simulink library "lib_energy_storage"  (Simulink 7.9)
settings: Solver=ode45  SolverMode=SingleTasking  StartTime=0.0  StopTime=10.0  RelTol=1e-3
undefined symbols (not defined in the file or in its folder): air_cp, amb_tmp, cyc_mph, enable_stop, ess_cap, ess_cap_scale, ess_cb, ess_cc, ess_coulombic_eff, ess_init_soc, ess_max_ah_cap, ess_max_p, ess_max_p_soc, ess_max_soc, ess_max_volts, ess_min_soc, ess_min_volts, ess_MMi, ess_MMo, ess_mod_airflow, ess_mod_cp, ess_mod_cpm, ess_mod_init_tmp, ess_module_mass, ess_module_num, ess_on, ess_parallel_mod_num, ess_r, ess_r_chg, ess_r_dis, ess_rc, ess_re, ess_res_scale_coef, ess_res_scale_fun, ess_rt, ess_set_tmp, ess_soc, ess_th_calc, ess_th_res, ess_th_res_off, ess_th_res_on, ess_tmp, ess_voc, fund_byu, fund_byuop, mc_min_volts, saber_air_temp, Saber_Battery_IO_File, saber_init_soc, saber_init_temp, saber_init_voc, saber_k_cb, saber_k_cc, saber_k_rc, saber_k_re, saber_k_rt, saber_k_soc, t_soc, time_step
libraries: lib_energy_storage x3
(part 1 of 3)
Description:
  | energy storage
settings Model: Creator=NREL  LastModifiedBy=mokeefe  ModifiedComment=mzolot -- Mon Apr 29 15:28:23 2002 -- Version 3.0107
settings Model: ModifiedHistory=|
  | mzolot -- Mon Apr 29 15:28:23 2002 -- Version 3.0107
  | 
  | 
  | mzolot -- Mon Apr 29 15:28:23 2002 -- Version 3.0107
  | 
  | 
  | mzolot -- Mon Apr 29 15:09:57 2002 -- Version 3.0106
  | 
  | 
  | mzolot -- Mon Apr 29 14:58:03 2002 -- Version 3.0105
  | 
  | 
  | mzolot -- Mon Apr 29 14:03:19 2002 -- Version 3.0104
  | 
  | 
  | mzolot -- Mon Apr 29 14:02:44 2002 -- Version 3.0103
  | 
  | 
  | mzolot -- Mon Apr 29 14:02:36 2002 -- Version 3.0102
  | 
  | 
  | mzolot -- Mon Apr 29 14:01:30 2002 -- Version 3.0101
  | 
  | 
  | mzolot -- Tue Apr 23 09:34:07 2002 -- Version 3.0100
  | 
  | 
  | mzolot -- Tue Apr 23 09:26:47 2002 -- Version 3.099
  | 
  | 
  | mzolot -- Tue Apr 23 09:26:41 2002 -- Version 3.098
  | 
  | 
  | mzolot -- Fri Apr 19 16:37:41 2002 -- Version 3.097
  | 
  | 
  | mzolot -- Fri Apr 19 11:13:38 2002 -- Version 3.096
  | 
  | 
  | mzolot -- Thu Apr 18 17:16:22 2002 -- Version 3.095
  | 
  | 
  | mokeefe -- Thu Apr 18 08:28:08 2002 -- Version 3.094
  | saving the model:
  | o "without the model browser open"
  | o with only top-level screen visible
  | o with "fit to view" enabled
  | o with "status bar" off and "toolbar" off
  | o with "prompt to update model history with each save" on
  | 
  | vjohnson -- Thu Jan 25 10:35:56 2001 -- Version 3.02
  | 
  | 
  | ssprik -- Wed Nov 01 15:28:33 2000 -- Version 3.01
  | enabled comment dialogue to prompt the person saving the model to add comments.

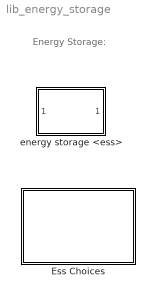
== system lib_energy_storage ==
  note: Energy Storage:
  Ess Choices : Subsystem
  energy storage <ess> : Subsystem  AncestorBlock=lib_energy_storage/Subsystem/energy storage <ess>
      mask Display: image(imread('bdi_ess.jpg'))

== system lib_energy_storage/Ess Choices ==
  note: Nnet
  note: Fundamental
  note: Saber Cosim
  Ultracapacitor  System : Subsystem
      mask Display: image(imread('bdi_ess.jpg'))
  energy storage <ess> : Subsystem
      mask Display: image(imread('bdi_ess.jpg'))
  energy storage <ess> RC : Subsystem
      mask Display: image(imread('bdi_ess.jpg'))
  energy storage <ess> nnet : Subsystem
      mask Display: image(imread('bdi_ess.jpg'))
  energy storage <ess> Saber : Subsystem
      mask Display: image(imread('bdi_ess.jpg'))
  energy storage <ess> fundamental model : Subsystem
      mask Display: image(imread('bdi_ess.jpg'))
  energy storage <ess> optima fundamental model : Subsystem
      mask Display: image(imread('bdi_ess.jpg'))
  ess config : Subsystem  BlockChoice="Ultracapacitor  System"
      settings: TemplateBlock=self  MemberBlocks="Ultracapacitor  System,energy storage <ess>,energy storage <ess> RC,energy storage <ess> nnet,energy storage <ess> Saber,energy storage <ess> fundamental model,energy storage <ess> optima fundamental model"

== system lib_energy_storage/energy storage <ess> ==
  power req'd into bus (W) : Inport
  ess config : Subsystem  BlockChoice="Ultracapacitor  System"
      settings: AttributesFormatString=%<BlockChoice>  TemplateBlock=lib_energy_storage/Ess Choices/ess config  MemberBlocks="Ultracapacitor  System,energy storage <ess>,energy storage <ess> RC,energy storage <ess> nnet,energy storage <ess> Saber,energy storage <ess> fundamental model,energy storage <ess> optima fundamental model"
  power available to bus (W) : Outport  InitialOutput=0
  wires:
  ess config/1(power available to bus (W)) -> power available to bus (W)/1
  power req'd into bus (W)/1 -> ess config/1(power req'd into bus (W))

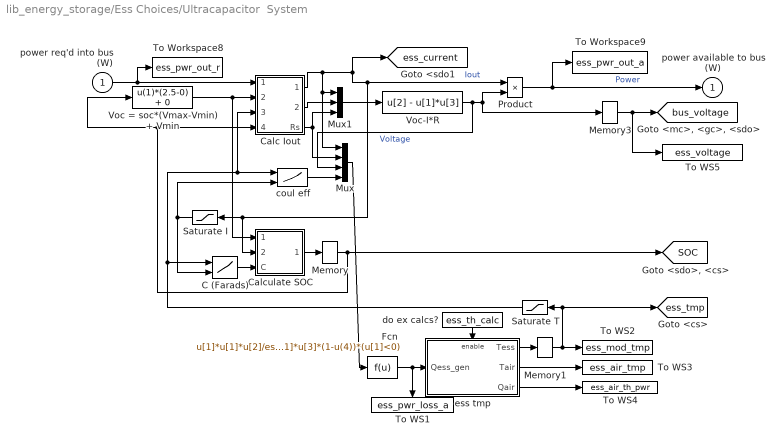
== system lib_energy_storage/Ess Choices/Ultracapacitor  System ==
  power req'd into bus (W) : Inport
  C (Farads) : Lookup2D  RowIndex=ess_tmp  ColumnIndex=ess_i  Table=ess_cap  SaturateOnIntegerOverflow=on  InputSameDT=on
  Calc Iout : Subsystem
  Calculate SOC : Subsystem
  Fcn : Fcn  Expr=u[1]*u[1]*u[2]/ess_parallel_mod_num*(u[1]>=0)+u[1]*u[1]*u(4)*u(4)*u[2]/ess_parallel_mod_num*(u[1]<0)-u[1]*u[3]*(1-u(4))*(u[1]<0)
  Memory : Memory  X0=ess_init_soc
  Memory1 : Memory  X0=ess_mod_init_tmp
  Memory3 : Memory  X0=(ess_init_soc*(2.5-0)+0)*ess_module_num
  Mux : Mux
  Mux1 : Mux  Inputs=3
  Product : Product  SaturateOnIntegerOverflow=on  RndMeth=Zero  InputSameDT=on  OutDataTypeStr=Inherit: Same as first input
  Saturate I : Saturate  UpperLimit=225  LowerLimit=-225
  Saturate T : Saturate  UpperLimit=40  LowerLimit=0
  To WS1 : ToWorkspace  VariableName=ess_pwr_loss_a
  To WS2 : ToWorkspace  VariableName=ess_mod_tmp
  To WS3 : ToWorkspace  VariableName=ess_air_tmp
  To WS4 : ToWorkspace  VariableName=ess_air_th_pwr
  To WS5 : ToWorkspace  VariableName=ess_voltage
  To Workspace8 : ToWorkspace  VariableName=ess_pwr_out_r  SampleTime=-1
  To Workspace9 : ToWorkspace  VariableName=ess_pwr_out_a  SampleTime=-1
  Voc = soc*(Vmax-Vmin) + Vmin : Fcn  Expr=u(1)*(2.5-0) + 0
  Voc-I*R : Fcn  Expr=u[2] - u[1]*u[3]
  coul eff : Lookup2D  RowIndex=ess_tmp  ColumnIndex=ess_i  Table=ess_coulombic_eff  SaturateOnIntegerOverflow=on  InputSameDT=on
  do ex calcs? : Constant  Value=ess_th_calc
  ess tmp : Subsystem  TreatAsAtomicUnit=on
  power available to bus (W) : Outport  InitialOutput=0
  tag scope: SOC=global, bus_voltage=global, ess_current=global, ess_tmp=global
  wires:
  power req'd into bus (W)/1 -> Calc Iout/1(Preq), To Workspace8/1
  Memory/1 -> [SOC], Voc = soc*(Vmax-Vmin) + Vmin/1, Calc Iout/4(SOC)
  Product/1 -> power available to bus (W)/1, To Workspace9/1  "Power"
  Calc Iout/1(Iout) -> Mux/1, Mux1/1, Product/1, Calculate SOC/2(Iout), Saturate I/1, [ess_current]  "Iout"
  coul eff/1 -> Mux/4
  Mux/1 -> Fcn/1
  Mux1/1 -> Voc-I*R/1
  Calc Iout/3(Rs) -> Mux/2, Mux1/3
  Fcn/1 -> ess tmp/1(Qess_gen), To WS1/1
  do ex calcs?/1 -> ess tmp/Enable
  ess tmp/1(Tess) -> Memory1/1
  ess tmp/2(Tair) -> To WS3/1
  Memory1/1 -> [ess_tmp], To WS2/1, Saturate T/1
  ess tmp/3(Qair) -> To WS4/1
  Voc-I*R/1 -> Product/2, Memory3/1, Mux/3  "Voltage"
  Memory3/1 -> [bus_voltage], To WS5/1
  Calculate SOC/1(SOC) -> Memory/1
  C (Farads)/1 -> Calculate SOC/3(C)
  Voc = soc*(Vmax-Vmin) + Vmin/1 -> Calc Iout/2(Voc), Calculate SOC/1(Voc)
  Saturate I/1 -> C (Farads)/2, coul eff/2
  Calc Iout/2(Voc*k) -> Mux1/2
  Saturate T/1 -> C (Farads)/1, coul eff/1, Calc Iout/3(tmp)

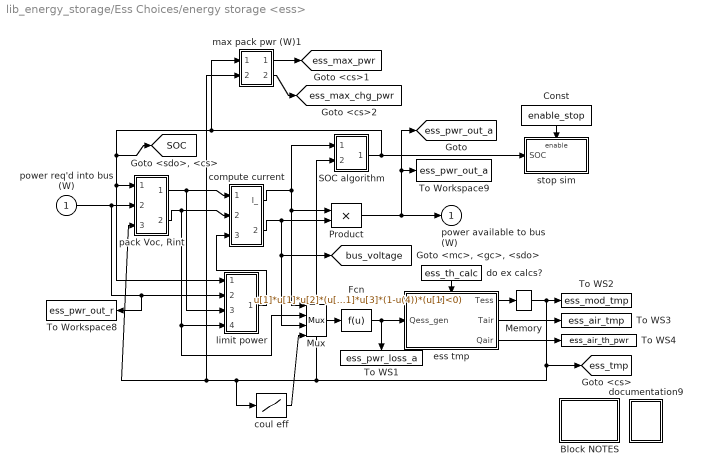
== system lib_energy_storage/Ess Choices/energy storage <ess> ==
  power req'd into bus (W) : Inport
  Block NOTES : Subsystem
      mask Display: disp('Block\nNOTES')
  Const : Constant  Value=enable_stop
  Fcn : Fcn  Expr=u[1]*u[1]*u[2]*(u[1]>=0)+u[1]*u[1]*u[2]*u(4)*u(4)*(u[1]<0)-u[1]*u[3]*(1-u(4))*(u[1]<0)
  Memory : Memory  X0=ess_mod_init_tmp
  Mux : Mux
  Product : Product  SaturateOnIntegerOverflow=on  RndMeth=Zero  InputSameDT=on  OutDataTypeStr=Inherit: Same as first input
  SOC algorithm : Subsystem
  To WS1 : ToWorkspace  VariableName=ess_pwr_loss_a
  To WS2 : ToWorkspace  VariableName=ess_mod_tmp
  To WS3 : ToWorkspace  VariableName=ess_air_tmp
  To WS4 : ToWorkspace  VariableName=ess_air_th_pwr
  To Workspace8 : ToWorkspace  VariableName=ess_pwr_out_r  SampleTime=-1
  To Workspace9 : ToWorkspace  VariableName=ess_pwr_out_a  SampleTime=-1
  compute current : Subsystem
  coul eff : Lookup  InputValues=ess_tmp  Table=ess_coulombic_eff  SaturateOnIntegerOverflow=on
  do ex calcs? : Constant  Value=ess_th_calc
  documentation9 : Subsystem
      settings: OpenFcn=web(['file:\\\' which('energy_storage.htm')]);
      mask Display: image(imread('doc_man.jpg'))
  ess tmp : Subsystem  TreatAsAtomicUnit=on
  limit power : Subsystem
  max pack pwr (W)1 : Subsystem
  "pack Voc, Rint" : Subsystem
  stop sim : Subsystem  TreatAsAtomicUnit=on
  power available to bus (W) : Outport  InitialOutput=0
  tag scope: SOC=global, bus_voltage=global, ess_max_chg_pwr=global, ess_max_pwr=global, ess_pwr_out_a=global, ess_tmp=global
  wires:
  compute current/2(V_) -> Product/2, Mux/3, [bus_voltage]
  Mux/1 -> Fcn/1
  power req'd into bus (W)/1 -> To Workspace8/1, limit power/2(Pbty), "pack Voc, Rint"/2(req'd battery power (W))
  compute current/1(I_) -> SOC algorithm/1((A)), Product/1, Mux/1
  Product/1 -> power available to bus (W)/1, To Workspace9/1, [ess_pwr_out_a]
  Fcn/1 -> To WS1/1, ess tmp/1(Qess_gen)
  do ex calcs?/1 -> ess tmp/Enable
  SOC algorithm/1(SOC1) -> stop sim/1(SOC), [SOC], "pack Voc, Rint"/1(SOC (prev)), limit power/1(SOC), max pack pwr (W)1/1(SOC)
  Const/1 -> stop sim/Enable
  "pack Voc, Rint"/2(pack resistance) -> compute current/2(Rint), limit power/4(Rint), Mux/2
  "pack Voc, Rint"/1(pack open- circuit voltage) -> compute current/1(Voc), limit power/3(Voc)
  limit power/1("Pbty, limited") -> compute current/3(limited output power (W))
  ess tmp/2(Tair) -> To WS3/1
  ess tmp/3(Qair) -> To WS4/1
  ess tmp/1(Tess) -> Memory/1
  coul eff/1 -> Mux/4
  max pack pwr (W)1/1(max ess discharge pwr) -> [ess_max_pwr]
  Memory/1 -> To WS2/1, SOC algorithm/2(tmp (C)), coul eff/1, "pack Voc, Rint"/3(mod tmp   (C)), max pack pwr (W)1/2(ess_mod_tmp), [ess_tmp]
  max pack pwr (W)1/2(max ess charge pwr) -> [ess_max_chg_pwr]

== system lib_energy_storage/Ess Choices/energy storage <ess> RC ==
  power req'd into bus (W) : Inport
  Allow simulation to stop based on  low SOC : Subsystem  TreatAsAtomicUnit=on
  Block NOTES : Subsystem
      mask Display: disp('Block\nNOTES')
  Const : Constant  Value=enable_stop
  Memory : Memory  X0=ess_mod_init_tmp
  Model Parameters : Subsystem
  RC model : Subsystem
  Thermal Model of Battery : Subsystem  TreatAsAtomicUnit=on
  To WS1 : ToWorkspace  VariableName=ess_pwr_loss_a
  To WS2 : ToWorkspace  VariableName=ess_mod_tmp
  To WS3 : ToWorkspace  VariableName=ess_air_tmp
  To WS4 : ToWorkspace  VariableName=ess_air_th_pwr
  To WS5 : ToWorkspace  VariableName=ess_voltage
  To Workspace8 : ToWorkspace  VariableName=ess_pwr_out_r  SampleTime=-1
  To Workspace9 : ToWorkspace  VariableName=ess_pwr_out_a  SampleTime=-1
  do ex calcs? : Constant  Value=ess_th_calc
  documentation9 : Subsystem
      settings: OpenFcn=web(['file:\\\' which('energy_storage.htm')]);
      mask Display: image(imread('doc_man.jpg'))
  power available to bus (W) : Outport  InitialOutput=0
  tag scope: SOC=global, bus_voltage=global, ess_tmp=global
  wires:
  RC model/1(Pavailable) -> To Workspace9/1, power available to bus (W)/1
  do ex calcs?/1 -> Thermal Model of Battery/Enable
  Thermal Model of Battery/2(Tair) -> To WS3/1
  Thermal Model of Battery/3(Qair) -> To WS4/1
  Thermal Model of Battery/1(Tess) -> Memory/1
  Memory/1 -> RC model/7(Ess Temp), Model Parameters/2(Ess Temp), [ess_tmp], To WS2/1
  Const/1 -> Allow simulation to stop based on  low SOC/Enable
  RC model/2(SOC) -> [SOC], Allow simulation to stop based on  low SOC/1(SOC), Model Parameters/1(SOC)
  RC model/4(Qess_gen) -> Thermal Model of Battery/1(Qess_gen), To WS1/1
  power req'd into bus (W)/1 -> To Workspace8/1, RC model/6(Preq), Model Parameters/3(Preq)
  Model Parameters/5(Rt) -> RC model/5(Rt)
  Model Parameters/4(Rc) -> RC model/4(Rc)
  Model Parameters/3(Re) -> RC model/3(Re)
  Model Parameters/2(Cc) -> RC model/2(Cc)
  Model Parameters/1(Cb) -> RC model/1(Cb)
  RC model/3(Vout) -> [bus_voltage], To WS5/1

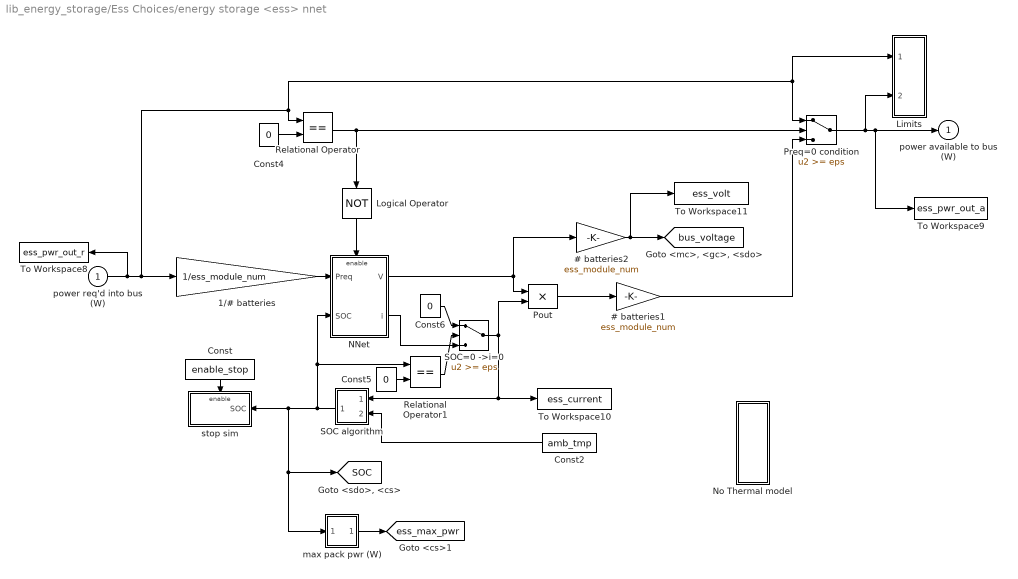
== system lib_energy_storage/Ess Choices/energy storage <ess> nnet ==
  power req'd into bus (W) : Inport
  # batteries1 : Gain  Gain=ess_module_num  SaturateOnIntegerOverflow=on  OutDataTypeStr=Inherit: Same as input  ParamDataTypeStr=Inherit: Same as input
  # batteries2 : Gain  Gain=ess_module_num  SaturateOnIntegerOverflow=on  OutDataTypeStr=Inherit: Same as input  ParamDataTypeStr=Inherit: Same as input
  1/# batteries : Gain  Gain=1/ess_module_num  SaturateOnIntegerOverflow=on  OutDataTypeStr=Inherit: Same as input  ParamDataTypeStr=Inherit: Same as input
  Const : Constant  Value=enable_stop
  Const2 : Constant  Value=amb_tmp
  Const4 : Constant  Value=0
  Const5 : Constant  Value=0
  Const6 : Constant  Value=0
  Limits : Subsystem
  Logical Operator : Logic  Operator=NOT  Inputs=1
  NNet : Subsystem  TreatAsAtomicUnit=on
  No Thermal model : Subsystem
  Pout : Product  SaturateOnIntegerOverflow=on  RndMeth=Zero  InputSameDT=on  OutDataTypeStr=Inherit: Same as first input
  Preq=0 condition : Switch  Threshold=eps  SaturateOnIntegerOverflow=on  InputSameDT=on
  Relational Operator : RelationalOperator  Operator===  InputSameDT=on
  Relational Operator1 : RelationalOperator  Operator===  InputSameDT=on
  SOC algorithm : Subsystem
  SOC=0 ->i=0 : Switch  Threshold=eps  SaturateOnIntegerOverflow=on  InputSameDT=on
  To Workspace10 : ToWorkspace  VariableName=ess_current  SampleTime=-1
  To Workspace11 : ToWorkspace  VariableName=ess_volt  SampleTime=-1
  To Workspace8 : ToWorkspace  VariableName=ess_pwr_out_r  SampleTime=-1
  To Workspace9 : ToWorkspace  VariableName=ess_pwr_out_a  SampleTime=-1
  max pack pwr (W) : Subsystem
  stop sim : Subsystem  TreatAsAtomicUnit=on
  power available to bus (W) : Outport  InitialOutput=0
  tag scope: SOC=global, bus_voltage=global, ess_max_pwr=global
  wires:
  SOC=0 ->i=0/1 -> Pout/2, To Workspace10/1, SOC algorithm/1((A))
  Relational Operator1/1 -> SOC=0 ->i=0/2
  Const5/1 -> Relational Operator1/2
  NNet/2(i) -> SOC=0 ->i=0/3
  Const6/1 -> SOC=0 ->i=0/1
  Const2/1 -> SOC algorithm/2(tmp (C))
  Preq=0 condition/1 -> Limits/2(power  available from battery), To Workspace9/1, power available to bus (W)/1
  # batteries1/1 -> Preq=0 condition/3
  # batteries2/1 -> To Workspace11/1, [bus_voltage]
  NNet/1(V) -> # batteries2/1, Pout/1
  Pout/1 -> # batteries1/1
  max pack pwr (W)/1(ess discharge pwr) -> [ess_max_pwr]
  Relational Operator/1 -> Logical Operator/1, Preq=0 condition/2
  Logical Operator/1 -> NNet/Enable
  Const4/1 -> Relational Operator/2
  1/# batteries/1 -> NNet/1(Preq)
  power req'd into bus (W)/1 -> Limits/1(power req), Preq=0 condition/1, Relational Operator/1, 1/# batteries/1, To Workspace8/1
  SOC algorithm/1(SOC1) -> Relational Operator1/1, NNet/2(SOC), max pack pwr (W)/1(SOC), [SOC], stop sim/1(SOC)
  Const/1 -> stop sim/Enable

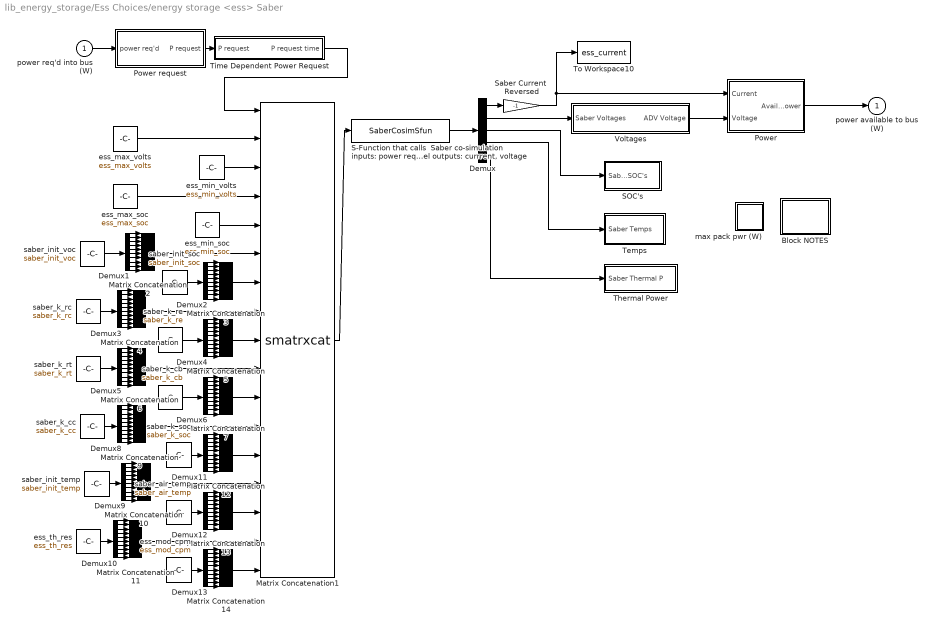
== system lib_energy_storage/Ess Choices/energy storage <ess> Saber ==
  power req'd into bus (W) : Inport
  Block NOTES : Subsystem
      mask Display: disp('Block\nNOTES')
  Demux : Demux  Outputs=[1 10 10 10 10]
  Demux{1..6,8..13} (12 alike) : Demux  Outputs=10
  Matrix Concatenation1 : S-Function  FunctionName=smatrxcat  Parameters=numInports,catMethod  EnableBusSupport=off  mask(Matrix Concatenation){numInports=17, catMethod=Horizontal}
      mask prompts: numInports "Number of inputs:"; catMethod "Concatenation method:"
      mask help: Perform horizontal or vertical concatenation. 1-D vector input signals are treated as column vectors, i.e., [Mx1] matrices. The output is always a matrix.
      mask init:
      | xy = matrxcatmask('icon');
      mask StyleString: edit,popup(Horizontal|Vertical)
      mask Display:
      | plot(xy.x,xy.y);
      | text(0.15,0.86,xy.label);
  Matrix Concatenation{2..7,9..14} (12 alike) : Concatenate  NumInputs=10  Mode=Multidimensional array  ConcatenateDimension=2
  Power : Subsystem
  Power request : Subsystem  AncestorBlock=lib_energy_storage/Ess Choices/energy storage <ess> Saber/Power request
  "S-Function that calls  Saber co-simulation inputs: power request load parameters outputs: accessory power model outputs: currrent, voltage" : S-Function  FunctionName=SaberCosimSfun  Parameters=strrep(which('advisor'),'advisor.m','tmp\'),time_step,Saber_Battery_IO_File  EnableBusSupport=off
  SOC's : Subsystem
  Saber Current  Reversed : Gain  Gain=-1  SaturateOnIntegerOverflow=on  OutDataTypeStr=Inherit: Same as input  ParamDataTypeStr=Inherit: Same as input
  Temps : Subsystem
  Thermal Power : Subsystem
  Time Dependent Power Request : Subsystem  AncestorBlock=lib_energy_storage/Ess Choices/energy storage <ess> Saber/Time Dependent Power Request
  To Workspace10 : ToWorkspace  VariableName=ess_current  SampleTime=-1
  Voltages : Subsystem
  ess_max_soc : Constant  Value=ess_max_soc
  ess_max_volts : Constant  Value=ess_max_volts
  ess_min_soc : Constant  Value=ess_min_soc
  ess_min_volts : Constant  Value=ess_min_volts
  ess_mod_cpm : Constant  Value=ess_mod_cpm
  ess_th_res : Constant  Value=ess_th_res
  max pack pwr (W) : Subsystem
  saber_air_temp : Constant  Value=saber_air_temp
  saber_init_soc : Constant  Value=saber_init_soc
  saber_init_temp : Constant  Value=saber_init_temp
  saber_init_voc : Constant  Value=saber_init_voc
  saber_k_cb : Constant  Value=saber_k_cb
  saber_k_cc : Constant  Value=saber_k_cc
  saber_k_rc : Constant  Value=saber_k_rc
  saber_k_re : Constant  Value=saber_k_re
  saber_k_rt : Constant  Value=saber_k_rt
  saber_k_soc : Constant  Value=saber_k_soc
  power available to bus (W) : Outport  InitialOutput=0
  wires:
  "S-Function that calls  Saber co-simulation inputs: power request load parameters outputs: accessory power model outputs: currrent, voltage"/1 -> Demux/1
  Demux/2 -> Voltages/1(Saber Voltages)
  Demux/4 -> Temps/1(Saber Temps)
  Demux/3 -> SOC's/1(Saber SOC's)
  Voltages/1(ADV Voltage) -> Power/2(Voltage)
  Power/1(Avail Power) -> power available to bus (W)/1
  Demux/1 -> Saber Current  Reversed/1
  Saber Current  Reversed/1 -> Power/1(Current), To Workspace10/1
  Demux/5 -> Thermal Power/1(Saber Thermal P)
  power req'd into bus (W)/1 -> Power request/1(power req'd)
  Matrix Concatenation1/1 -> "S-Function that calls  Saber co-simulation inputs: power request load parameters outputs: accessory power model outputs: currrent, voltage"/1
  Time Dependent Power Request/1(P request time) -> Matrix Concatenation1/1
  ess_max_volts/1 -> Matrix Concatenation1/2
  ess_min_volts/1 -> Matrix Concatenation1/3
  ess_max_soc/1 -> Matrix Concatenation1/4
  ess_min_soc/1 -> Matrix Concatenation1/5
  Demux1/1 -> Matrix Concatenation2/1
  Demux1/2 -> Matrix Concatenation2/2
  Demux1/3 -> Matrix Concatenation2/3
  Demux1/4 -> Matrix Concatenation2/4
  Demux1/5 -> Matrix Concatenation2/5
  Demux1/6 -> Matrix Concatenation2/6
  Demux1/7 -> Matrix Concatenation2/7
  Demux1/8 -> Matrix Concatenation2/8
  Demux1/9 -> Matrix Concatenation2/9
  Demux1/10 -> Matrix Concatenation2/10
  saber_init_soc/1 -> Demux2/1
  Demux2/1 -> Matrix Concatenation3/1
  Demux2/2 -> Matrix Concatenation3/2
  Demux2/3 -> Matrix Concatenation3/3
  Demux2/4 -> Matrix Concatenation3/4
  Demux2/5 -> Matrix Concatenation3/5
  Demux2/6 -> Matrix Concatenation3/6
  Demux2/7 -> Matrix Concatenation3/7
  Demux2/8 -> Matrix Concatenation3/8
  Demux2/9 -> Matrix Concatenation3/9
  Demux2/10 -> Matrix Concatenation3/10
  saber_k_rc/1 -> Demux3/1
  Demux3/1 -> Matrix Concatenation4/1
  Demux3/2 -> Matrix Concatenation4/2
  Demux3/3 -> Matrix Concatenation4/3
  Demux3/4 -> Matrix Concatenation4/4
  Demux3/5 -> Matrix Concatenation4/5
  Demux3/6 -> Matrix Concatenation4/6
  Demux3/7 -> Matrix Concatenation4/7
  Demux3/8 -> Matrix Concatenation4/8
  Demux3/9 -> Matrix Concatenation4/9
  Demux3/10 -> Matrix Concatenation4/10
  saber_k_re/1 -> Demux4/1
  Demux4/1 -> Matrix Concatenation5/1
  Demux4/2 -> Matrix Concatenation5/2
  Demux4/3 -> Matrix Concatenation5/3
  Demux4/4 -> Matrix Concatenation5/4
  Demux4/5 -> Matrix Concatenation5/5
  Demux4/6 -> Matrix Concatenation5/6
  Demux4/7 -> Matrix Concatenation5/7
  Demux4/8 -> Matrix Concatenation5/8
  Demux4/9 -> Matrix Concatenation5/9
  Demux4/10 -> Matrix Concatenation5/10
  Demux5/1 -> Matrix Concatenation6/1
  Demux5/2 -> Matrix Concatenation6/2
  Demux5/3 -> Matrix Concatenation6/3
  Demux5/4 -> Matrix Concatenation6/4
  Demux5/5 -> Matrix Concatenation6/5
  Demux5/6 -> Matrix Concatenation6/6
  Demux5/7 -> Matrix Concatenation6/7
  Demux5/8 -> Matrix Concatenation6/8
  Demux5/9 -> Matrix Concatenation6/9
  Demux5/10 -> Matrix Concatenation6/10
  saber_k_cb/1 -> Demux6/1
  Demux6/1 -> Matrix Concatenation7/1
  Demux6/2 -> Matrix Concatenation7/2
  Demux6/3 -> Matrix Concatenation7/3
  Demux6/4 -> Matrix Concatenation7/4
  Demux6/5 -> Matrix Concatenation7/5
  Demux6/6 -> Matrix Concatenation7/6
  Demux6/7 -> Matrix Concatenation7/7
  Demux6/8 -> Matrix Concatenation7/8
  Demux6/9 -> Matrix Concatenation7/9
  Demux6/10 -> Matrix Concatenation7/10
  saber_k_rt/1 -> Demux5/1
  Matrix Concatenation2/1 -> Matrix Concatenation1/6
  saber_init_voc/1 -> Demux1/1
  Matrix Concatenation3/1 -> Matrix Concatenation1/7
  Matrix Concatenation4/1 -> Matrix Concatenation1/8
  Matrix Concatenation6/1 -> Matrix Concatenation1/10
  Matrix Concatenation7/1 -> Matrix Concatenation1/11
  Matrix Concatenation5/1 -> Matrix Concatenation1/9
  saber_k_cc/1 -> Demux8/1
  Demux8/1 -> Matrix Concatenation9/1
  Demux8/2 -> Matrix Concatenation9/2
  Demux8/3 -> Matrix Concatenation9/3
  Demux8/4 -> Matrix Concatenation9/4
  Demux8/5 -> Matrix Concatenation9/5
  Demux8/6 -> Matrix Concatenation9/6
  Demux8/7 -> Matrix Concatenation9/7
  Demux8/8 -> Matrix Concatenation9/8
  Demux8/9 -> Matrix Concatenation9/9
  Demux8/10 -> Matrix Concatenation9/10
  saber_init_temp/1 -> Demux9/1
  Demux9/1 -> Matrix Concatenation10/1
  Demux9/2 -> Matrix Concatenation10/2
  Demux9/3 -> Matrix Concatenation10/3
  Demux9/4 -> Matrix Concatenation10/4
  Demux9/5 -> Matrix Concatenation10/5
  Demux9/6 -> Matrix Concatenation10/6
  Demux9/7 -> Matrix Concatenation10/7
  Demux9/8 -> Matrix Concatenation10/8
  Demux9/9 -> Matrix Concatenation10/9
  Demux9/10 -> Matrix Concatenation10/10
  ess_th_res/1 -> Demux10/1
  Demux10/1 -> Matrix Concatenation11/1
  Demux10/2 -> Matrix Concatenation11/2
  Demux10/3 -> Matrix Concatenation11/3
  Demux10/4 -> Matrix Concatenation11/4
  Demux10/5 -> Matrix Concatenation11/5
  Demux10/6 -> Matrix Concatenation11/6
  Demux10/7 -> Matrix Concatenation11/7
  Demux10/8 -> Matrix Concatenation11/8
  Demux10/9 -> Matrix Concatenation11/9
  Demux10/10 -> Matrix Concatenation11/10
  saber_k_soc/1 -> Demux11/1
  Demux11/1 -> Matrix Concatenation12/1
  Demux11/2 -> Matrix Concatenation12/2
  Demux11/3 -> Matrix Concatenation12/3
  Demux11/4 -> Matrix Concatenation12/4
  Demux11/5 -> Matrix Concatenation12/5
  Demux11/6 -> Matrix Concatenation12/6
  Demux11/7 -> Matrix Concatenation12/7
  Demux11/8 -> Matrix Concatenation12/8
  Demux11/9 -> Matrix Concatenation12/9
  Demux11/10 -> Matrix Concatenation12/10
  Matrix Concatenation12/1 -> Matrix Concatenation1/13
  saber_air_temp/1 -> Demux12/1
  Demux12/1 -> Matrix Concatenation13/1
  Demux12/2 -> Matrix Concatenation13/2
  Demux12/3 -> Matrix Concatenation13/3
  Demux12/4 -> Matrix Concatenation13/4
  Demux12/5 -> Matrix Concatenation13/5
  Demux12/6 -> Matrix Concatenation13/6
  Demux12/7 -> Matrix Concatenation13/7
  Demux12/8 -> Matrix Concatenation13/8
  Demux12/9 -> Matrix Concatenation13/9
  Demux12/10 -> Matrix Concatenation13/10
  Matrix Concatenation13/1 -> Matrix Concatenation1/15
  ess_mod_cpm/1 -> Demux13/1
  Demux13/1 -> Matrix Concatenation14/1
  Demux13/2 -> Matrix Concatenation14/2
  Demux13/3 -> Matrix Concatenation14/3
  Demux13/4 -> Matrix Concatenation14/4
  Demux13/5 -> Matrix Concatenation14/5
  Demux13/6 -> Matrix Concatenation14/6
  Matrix Concatenation14/1 -> Matrix Concatenation1/17
  Matrix Concatenation9/1 -> Matrix Concatenation1/12
  Matrix Concatenation10/1 -> Matrix Concatenation1/14
  Matrix Concatenation11/1 -> Matrix Concatenation1/16
  Demux13/7 -> Matrix Concatenation14/7
  Demux13/9 -> Matrix Concatenation14/9
  Demux13/8 -> Matrix Concatenation14/8
  Demux13/10 -> Matrix Concatenation14/10
  Power request/1(P request) -> Time Dependent Power Request/1(P request)

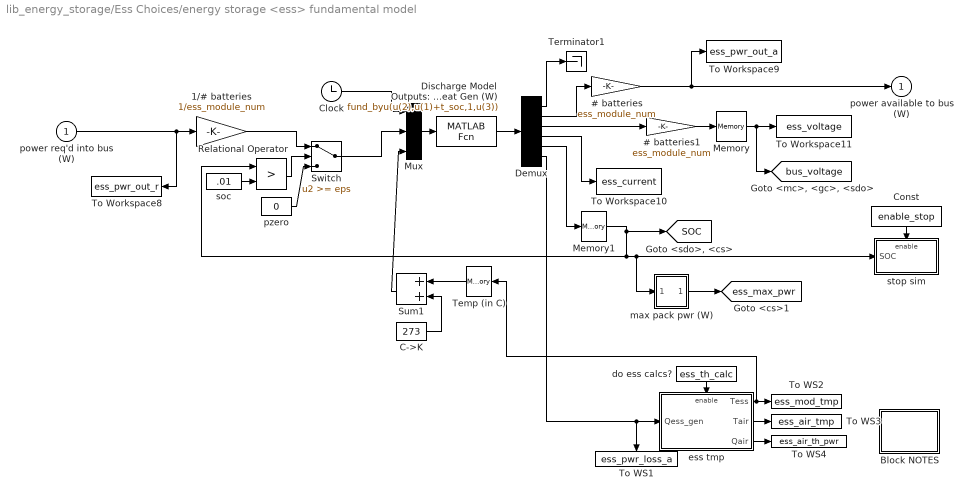
== system lib_energy_storage/Ess Choices/energy storage <ess> fundamental model ==
  power req'd into bus (W) : Inport
  # batteries : Gain  Gain=ess_module_num  SaturateOnIntegerOverflow=on  OutDataTypeStr=Inherit: Same as input  ParamDataTypeStr=Inherit: Same as input
  # batteries1 : Gain  Gain=ess_module_num  SaturateOnIntegerOverflow=on  OutDataTypeStr=Inherit: Same as input  ParamDataTypeStr=Inherit: Same as input
  1/# batteries : Gain  Gain=1/ess_module_num  SaturateOnIntegerOverflow=on  OutDataTypeStr=Inherit: Same as input  ParamDataTypeStr=Inherit: Same as input
  Block NOTES : Subsystem
      mask Display: disp('Block\nNOTES')
  C->K : Constant  Value=273
  Clock : Clock
  Const : Constant  Value=enable_stop
  Demux : Demux  Outputs=6
  Discharge Model Outputs: Preq(W) Pavail (W) Voltage (V) Current (A) SOC Heat Gen (W) : MATLABFcn  MATLABFcn=fund_byu(u(2),u(1)+t_soc,1,u(3))
  Memory : Memory  X0=12*ess_module_num
  Memory1 : Memory  X0=ess_init_soc
  Mux : Mux  Inputs=3
  Relational Operator : RelationalOperator  Operator=>  InputSameDT=on
  Sum1 : Sum  SaturateOnIntegerOverflow=on  InputSameDT=on  OutDataTypeStr=Inherit: Same as first input
  Switch : Switch  Threshold=eps  SaturateOnIntegerOverflow=on  InputSameDT=on
  Temp (in C) : Memory  X0=amb_tmp
  Terminator1 : Terminator
  To WS1 : ToWorkspace  VariableName=ess_pwr_loss_a
      settings: MaxDataPoints=50000
  To WS2 : ToWorkspace  VariableName=ess_mod_tmp
      settings: MaxDataPoints=50000
  To WS3 : ToWorkspace  VariableName=ess_air_tmp
      settings: MaxDataPoints=50000
  To WS4 : ToWorkspace  VariableName=ess_air_th_pwr
      settings: MaxDataPoints=50000
  To Workspace10 : ToWorkspace  VariableName=ess_current  SampleTime=-1
  To Workspace11 : ToWorkspace  VariableName=ess_voltage  SampleTime=-1
  To Workspace8 : ToWorkspace  VariableName=ess_pwr_out_r  SampleTime=-1
  To Workspace9 : ToWorkspace  VariableName=ess_pwr_out_a  SampleTime=-1
  do ess calcs? : Constant  Value=ess_th_calc
  ess tmp : Subsystem  TreatAsAtomicUnit=on
  max pack pwr (W) : Subsystem
  pzero : Constant  Value=0
  soc : Constant  Value=.01
  stop sim : Subsystem  TreatAsAtomicUnit=on
  power available to bus (W) : Outport  InitialOutput=0
  tag scope: SOC=global, bus_voltage=global, ess_max_pwr=global
  wires:
  ess tmp/1(Tess) -> Temp (in C)/1, To WS2/1
  ess tmp/3(Qair) -> To WS4/1
  ess tmp/2(Tair) -> To WS3/1
  do ess calcs?/1 -> ess tmp/Enable
  Demux/6 -> To WS1/1, ess tmp/1(Qess_gen)
  max pack pwr (W)/1(ess discharge pwr) -> [ess_max_pwr]
  Const/1 -> stop sim/Enable
  Sum1/1 -> Mux/3
  C->K/1 -> Sum1/2
  Temp (in C)/1 -> Sum1/1
  Memory1/1 -> [SOC], max pack pwr (W)/1(SOC), stop sim/1(SOC), Relational Operator/1
  Memory/1 -> [bus_voltage], To Workspace11/1
  Demux/3 -> # batteries1/1
  # batteries1/1 -> Memory/1
  # batteries/1 -> power available to bus (W)/1, To Workspace9/1
  Demux/1 -> Terminator1/1
  Switch/1 -> Mux/2
  1/# batteries/1 -> Switch/1
  soc/1 -> Relational Operator/2
  Relational Operator/1 -> Switch/2
  pzero/1 -> Switch/3
  power req'd into bus (W)/1 -> 1/# batteries/1, To Workspace8/1
  Clock/1 -> Mux/1
  Demux/2 -> # batteries/1
  Demux/4 -> To Workspace10/1
  Demux/5 -> Memory1/1
  Discharge Model Outputs: Preq(W) Pavail (W) Voltage (V) Current (A) SOC Heat Gen (W)/1 -> Demux/1
  Mux/1 -> Discharge Model Outputs: Preq(W) Pavail (W) Voltage (V) Current (A) SOC Heat Gen (W)/1

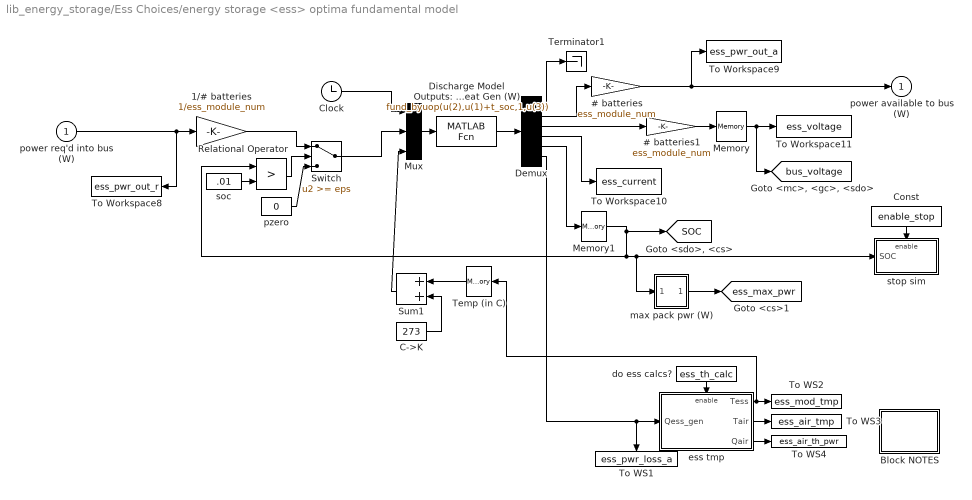
== system lib_energy_storage/Ess Choices/energy storage <ess> optima fundamental model ==
  power req'd into bus (W) : Inport
  # batteries : Gain  Gain=ess_module_num  SaturateOnIntegerOverflow=on  OutDataTypeStr=Inherit: Same as input  ParamDataTypeStr=Inherit: Same as input
  # batteries1 : Gain  Gain=ess_module_num  SaturateOnIntegerOverflow=on  OutDataTypeStr=Inherit: Same as input  ParamDataTypeStr=Inherit: Same as input
  1/# batteries : Gain  Gain=1/ess_module_num  SaturateOnIntegerOverflow=on  OutDataTypeStr=Inherit: Same as input  ParamDataTypeStr=Inherit: Same as input
  Block NOTES : Subsystem
      mask Display: disp('Block\nNOTES')
  C->K : Constant  Value=273
  Clock : Clock
  Const : Constant  Value=enable_stop
  Demux : Demux  Outputs=6
  Discharge Model Outputs: Preq(W) Pavail (W) Voltage (V) Current (A) SOC Heat Gen (W) : MATLABFcn  MATLABFcn=fund_byuop(u(2),u(1)+t_soc,1,u(3))
  Memory : Memory  X0=12*ess_module_num
  Memory1 : Memory  X0=ess_init_soc
  Mux : Mux  Inputs=3
  Relational Operator : RelationalOperator  Operator=>  InputSameDT=on
  Sum1 : Sum  SaturateOnIntegerOverflow=on  InputSameDT=on  OutDataTypeStr=Inherit: Same as first input
  Switch : Switch  Threshold=eps  SaturateOnIntegerOverflow=on  InputSameDT=on
  Temp (in C) : Memory  X0=amb_tmp
  Terminator1 : Terminator
  To WS1 : ToWorkspace  VariableName=ess_pwr_loss_a
      settings: MaxDataPoints=50000
  To WS2 : ToWorkspace  VariableName=ess_mod_tmp
      settings: MaxDataPoints=50000
  To WS3 : ToWorkspace  VariableName=ess_air_tmp
      settings: MaxDataPoints=50000
  To WS4 : ToWorkspace  VariableName=ess_air_th_pwr
      settings: MaxDataPoints=50000
  To Workspace10 : ToWorkspace  VariableName=ess_current  SampleTime=-1
  To Workspace11 : ToWorkspace  VariableName=ess_voltage  SampleTime=-1
  To Workspace8 : ToWorkspace  VariableName=ess_pwr_out_r  SampleTime=-1
  To Workspace9 : ToWorkspace  VariableName=ess_pwr_out_a  SampleTime=-1
  do ess calcs? : Constant  Value=ess_th_calc
  ess tmp : Subsystem  TreatAsAtomicUnit=on
  max pack pwr (W) : Subsystem
  pzero : Constant  Value=0
  soc : Constant  Value=.01
  stop sim : Subsystem  TreatAsAtomicUnit=on
  power available to bus (W) : Outport  InitialOutput=0
  tag scope: SOC=global, bus_voltage=global, ess_max_pwr=global
  wires:
  ess tmp/1(Tess) -> Temp (in C)/1, To WS2/1
  ess tmp/3(Qair) -> To WS4/1
  ess tmp/2(Tair) -> To WS3/1
  do ess calcs?/1 -> ess tmp/Enable
  Demux/6 -> To WS1/1, ess tmp/1(Qess_gen)
  max pack pwr (W)/1(ess discharge pwr) -> [ess_max_pwr]
  Const/1 -> stop sim/Enable
  Sum1/1 -> Mux/3
  C->K/1 -> Sum1/2
  Temp (in C)/1 -> Sum1/1
  Memory1/1 -> [SOC], max pack pwr (W)/1(SOC), stop sim/1(SOC), Relational Operator/1
  Memory/1 -> [bus_voltage], To Workspace11/1
  Demux/3 -> # batteries1/1
  # batteries1/1 -> Memory/1
  # batteries/1 -> power available to bus (W)/1, To Workspace9/1
  Demux/1 -> Terminator1/1
  Switch/1 -> Mux/2
  1/# batteries/1 -> Switch/1
  soc/1 -> Relational Operator/2
  Relational Operator/1 -> Switch/2
  pzero/1 -> Switch/3
  power req'd into bus (W)/1 -> 1/# batteries/1, To Workspace8/1
  Clock/1 -> Mux/1
  Demux/2 -> # batteries/1
  Demux/4 -> To Workspace10/1
  Demux/5 -> Memory1/1
  Discharge Model Outputs: Preq(W) Pavail (W) Voltage (V) Current (A) SOC Heat Gen (W)/1 -> Demux/1
  Mux/1 -> Discharge Model Outputs: Preq(W) Pavail (W) Voltage (V) Current (A) SOC Heat Gen (W)/1

== system lib_energy_storage/Ess Choices/ess config ==
  power req'd into bus (W) : Inport
  Ultracapacitor  System : lib_energy_storage/Subsystem/Ultracapacitor  System
      settings: RTWFcnNameOpts=Auto  RTWFileNameOpts=Auto
  power available to bus (W) : Outport

== system lib_energy_storage/energy storage <ess>/ess config ==
  power req'd into bus (W) : Inport
  Ultracapacitor  System : lib_energy_storage/Subsystem/Ultracapacitor  System
      settings: RTWFcnNameOpts=Auto  RTWFileNameOpts=Auto
  power available to bus (W) : Outport

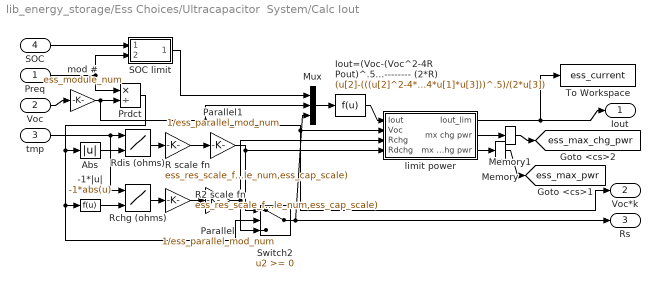
== system lib_energy_storage/Ess Choices/Ultracapacitor  System/Calc Iout ==
  Preq : Inport
  Voc : Inport  Port=2
  tmp : Inport  Port=3
  SOC : Inport  Port=4
  -1*|u| : Fcn  Expr=-1*abs(u)
  Abs : Abs  SaturateOnIntegerOverflow=on
  Iout=(Voc-(Voc^2-4RPout)^.5)        ----------------------------- (2*R) : Fcn  Expr=(u[2]-(((u[2]^2-4*u[1]*u[3])>0)*(u[2]^2-4*u[1]*u[3]))^.5)/(2*u[3])
  Memory : Memory
  Memory1 : Memory
  Mux : Mux  Inputs=3
  Parallel : Gain  Gain=1/ess_parallel_mod_num  SaturateOnIntegerOverflow=on  OutDataTypeStr=Inherit: Same as input  ParamDataTypeStr=Inherit: Same as input
  Parallel1 : Gain  Gain=1/ess_parallel_mod_num  SaturateOnIntegerOverflow=on  OutDataTypeStr=Inherit: Same as input  ParamDataTypeStr=Inherit: Same as input
  Prdct : Product  Inputs=*/  SaturateOnIntegerOverflow=on  RndMeth=Zero  InputSameDT=on  OutDataTypeStr=Inherit: Same as first input
  R scale fn : Gain  Gain=ess_res_scale_fun(ess_res_scale_coef,ess_module_num,ess_cap_scale)  SaturateOnIntegerOverflow=on  OutDataTypeStr=Inherit: Same as input  ParamDataTypeStr=Inherit: Same as input
  R2 scale fn : Gain  Gain=ess_res_scale_fun(ess_res_scale_coef,ess_module_num,ess_cap_scale)  SaturateOnIntegerOverflow=on  OutDataTypeStr=Inherit: Same as input  ParamDataTypeStr=Inherit: Same as input
  Rchg (ohms) : Lookup2D  RowIndex=ess_tmp  ColumnIndex=ess_i  Table=ess_r  SaturateOnIntegerOverflow=on  InputSameDT=on
  Rdis (ohms) : Lookup2D  RowIndex=ess_tmp  ColumnIndex=ess_i  Table=ess_r  SaturateOnIntegerOverflow=on  InputSameDT=on
  SOC limit : Subsystem
  Switch2 : Switch  SaturateOnIntegerOverflow=on  InputSameDT=on
  To Workspace : ToWorkspace  VariableName=ess_current  SampleTime=-1
  limit power : Subsystem
  mod # : Gain  Gain=ess_module_num  SaturateOnIntegerOverflow=on  OutDataTypeStr=Inherit: Same as input  ParamDataTypeStr=Inherit: Same as input
  Iout : Outport
  Voc*k : Outport  Port=2
  Rs : Outport  Port=3
  tag scope: ess_max_chg_pwr=global, ess_max_pwr=global
  wires:
  Preq/1 -> Prdct/1, SOC limit/2(Pbty)
  SOC/1 -> SOC limit/1(SOC)
  Mux/1 -> Iout=(Voc-(Voc^2-4RPout)^.5)        ----------------------------- (2*R)/1
  Rdis (ohms)/1 -> R scale fn/1
  R scale fn/1 -> Parallel1/1
  Rchg (ohms)/1 -> R2 scale fn/1
  Prdct/1 -> Abs/1, Switch2/2, -1*|u|/1
  Abs/1 -> Rdis (ohms)/2
  -1*|u|/1 -> Rchg (ohms)/2
  R2 scale fn/1 -> Parallel/1
  SOC limit/1("Pbty, limited") -> Mux/1
  Switch2/1 -> Rs/1, Mux/3
  limit power/1(Iout_lim) -> Iout/1, To Workspace/1
  Iout=(Voc-(Voc^2-4RPout)^.5)        ----------------------------- (2*R)/1 -> limit power/1(Iout)
  Voc/1 -> mod #/1
  mod #/1 -> Mux/2, limit power/2(Voc), Voc*k/1, Prdct/2
  tmp/1 -> Rdis (ohms)/1, Rchg (ohms)/1
  Memory/1 -> [ess_max_pwr]
  limit power/3(mx dchg pwr) -> Memory/1
  limit power/2(mx chg pwr) -> Memory1/1
  Memory1/1 -> [ess_max_chg_pwr]
  Parallel1/1 -> Switch2/1, limit power/4(Rdchg)
  Parallel/1 -> Switch2/3, limit power/3(Rchg)

== system lib_energy_storage/Ess Choices/Ultracapacitor  System/Calculate SOC ==
  Voc : Inport
  Iout : Inport  Port=2
  C : Inport  Port=3
  Clock : Clock
  Gain : Gain  Gain=ess_parallel_mod_num  SaturateOnIntegerOverflow=on  OutDataTypeStr=Inherit: Same as input  ParamDataTypeStr=Inherit: Same as input
  Memory : Memory
  Mux1 : Mux
  Saturation : Saturate  UpperLimit=1  LowerLimit=0
  Soc = (Voc(n+1)-Vmin)/(Vmax-Vmin) : Fcn  Expr=(u(1)-0)/(2.5-0)
  Sum : Sum  Inputs=|+-  SaturateOnIntegerOverflow=on  InputSameDT=on  OutDataTypeStr=Inherit: Same as first input
  Voc (n+1) = Voc(n) - I*(dt)/C : Fcn  Expr=(u(1) - u(2)*u(4)/u(3))
  SOC : Outport
  wires:
  Voc/1 -> Mux1/1
  Mux1/1 -> Voc (n+1) = Voc(n) - I*(dt)/C/1
  Iout/1 -> Mux1/2
  Voc (n+1) = Voc(n) - I*(dt)/C/1 -> Soc = (Voc(n+1)-Vmin)/(Vmax-Vmin)/1
  C/1 -> Gain/1
  Soc = (Voc(n+1)-Vmin)/(Vmax-Vmin)/1 -> Saturation/1
  Memory/1 -> Sum/2
  Clock/1 -> Memory/1, Sum/1
  Sum/1 -> Mux1/4
  Saturation/1 -> SOC/1
  Gain/1 -> Mux1/3

== system lib_energy_storage/Ess Choices/Ultracapacitor  System/ess tmp ==
  Qess_gen : Inport
  Enable : EnablePort  StatesWhenEnabling=reset
  #of mods : Gain  Gain=ess_module_num  SaturateOnIntegerOverflow=on  OutDataTypeStr=Inherit: Same as input  ParamDataTypeStr=Inherit: Same as input
  1/#of mods : Gain  Gain=1/ess_module_num  SaturateOnIntegerOverflow=on  OutDataTypeStr=Inherit: Same as input  ParamDataTypeStr=Inherit: Same as input
  1/mcp : Gain  Gain=1/(ess_module_mass*ess_mod_cp)  SaturateOnIntegerOverflow=on  OutDataTypeStr=Inherit: Same as input  ParamDataTypeStr=Inherit: Same as input
  Block NOTES : Subsystem
      mask Display: disp('Block\nNOTES')
  Memory : Memory  X0=cyc_mph(1,2)*.447
  Memory1 : Memory  X0=cyc_mph(1,2)*.447
  Mux20 : Mux  Inputs=3
  Qc : Sum  SaturateOnIntegerOverflow=on  InputSameDT=on  OutDataTypeStr=Inherit: Same as first input
  Qess_case : Fcn  Expr=(u(2) - u(1))/u(3)
  Saturation3 : Saturate  UpperLimit=1  LowerLimit=0
  Tair,ave : Subsystem  TreatAsAtomicUnit=on
  Tess2 : Integrator  InitialCondition=ess_mod_init_tmp
  thermostat : Fcn  Expr=u(1) - ess_set_tmp
  Tess : Outport  InitialOutput=0
  Tair : Outport  Port=2
  Qair : Outport  Port=3  OutputWhenDisabled=reset  InitialOutput=0
  wires:
  Qc/1 -> 1/mcp/1
  Qess_case/1 -> Qc/1, Memory/1, #of mods/1
  1/mcp/1 -> Tess2/1
  Tess2/1 -> Tess/1, Mux20/1, thermostat/1
  Qess_gen/1 -> 1/#of mods/1
  1/#of mods/1 -> Qc/2
  thermostat/1 -> Saturation3/1
  Saturation3/1 -> Memory1/1
  Memory1/1 -> Tair,ave/Enable
  Memory/1 -> Tair,ave/1(Qess_case)
  #of mods/1 -> Qair/1
  Mux20/1 -> Qess_case/1
  Tair,ave/2(Th Res) -> Mux20/3
  Tair,ave/1(Tair_ave) -> Mux20/2, Tair/1

== system lib_energy_storage/Ess Choices/energy storage <ess>/Block NOTES ==
  note: This block models the energy storage system as an SOC-dependent voltage
      | in series with an SOC- and current direction-dependent internal resistance.
      | SOC is computed assuming that A-h capacity is constant, but limited
      | such that a minimum voltage is never exceeded (replacing the
      | previous Peukert relationship which underpredicted battery capacity).
      |
      | Discharge power is limited here so as not to bring the bus (battery pack) voltage below
      | the minimum controller voltage or the minimum battery voltage and so as to allow
      | the solution of the quadratic eq'n for discharge current.
      |
      | Charge current is limited to ensure the voltage does not exceed a maximum
      | voltage
      |
      | Positive current is discharge current in the convention used here.
      | Power loss is computed as I*R+losses due to Coulombic (in)efficiency.
      |
      | Thermal modeling of the battery performance is modeled in the
      | OCV, Rint, and capacity.

== system lib_energy_storage/Ess Choices/energy storage <ess>/SOC algorithm ==
  note: SOC=(Max Ah capacity-Ah used)/Max Ah capacity
  (A) : Inport
  tmp (C) : Inport  Port=2
  (sec->hrs) : Gain  Gain=1/3600  SaturateOnIntegerOverflow=on  OutDataTypeStr=Inherit: Same as input  ParamDataTypeStr=Inherit: Same as input
  0 <= SOC <= 1 : Saturate  UpperLimit=1  LowerLimit=0
  A-h remaining : Sum  Inputs=-+  SaturateOnIntegerOverflow=on  InputSameDT=on  OutDataTypeStr=Inherit: Same as first input
  Ah used : Integrator  InitialConditionSource=external  InitialCondition=(1-ess_init_soc)*ess_max_ah_cap
  Fcn : Fcn  Expr=1/u
  Fcn1 : Fcn  Expr=(1-ess_init_soc)*u
  SOC : Product  SaturateOnIntegerOverflow=on  RndMeth=Zero  InputSameDT=on  OutDataTypeStr=Inherit: Same as first input
  Switch : Switch  SaturateOnIntegerOverflow=on  InputSameDT=on
  adjusted A : Product  SaturateOnIntegerOverflow=on  RndMeth=Zero  InputSameDT=on  OutDataTypeStr=Inherit: Same as first input
  coul eff : Lookup  InputValues=ess_tmp  Table=ess_coulombic_eff  SaturateOnIntegerOverflow=on
  max cap : Lookup  InputValues=ess_tmp  Table=ess_max_ah_cap*ess_cap_scale  SaturateOnIntegerOverflow=on
  SOC1 : Outport  InitialOutput=0
  wires:
  Fcn1/1 -> Ah used/2
  max cap/1 -> Fcn1/1, Fcn/1, A-h remaining/2
  adjusted A/1 -> Switch/3
  coul eff/1 -> adjusted A/2
  tmp (C)/1 -> coul eff/1, max cap/1
  0 <= SOC <= 1/1 -> SOC1/1
  A-h remaining/1 -> SOC/1
  SOC/1 -> 0 <= SOC <= 1/1
  Fcn/1 -> SOC/2
  Ah used/1 -> A-h remaining/1
  (sec->hrs)/1 -> Ah used/1
  Switch/1 -> (sec->hrs)/1
  (A)/1 -> adjusted A/1, Switch/1, Switch/2

== system lib_energy_storage/Ess Choices/energy storage <ess>/compute current ==
  Voc : Inport
  Rint : Inport  Port=2
  limited output power (W) : Inport  Port=3
  Ibty=(Voc-(Voc^2-4RPbty)^.5)        ----------------------------- (2*R) : Fcn  Expr=(u[2]-(u[2]^2-4*u[1]*u[3])^.5)/(2*u[3])
  Logical Operator1 : Logic  Operator=NOT  Inputs=1
  Mux3 : Mux  Inputs=3
  Mux4 : Mux  Inputs=3
  Mux5 : Mux  Inputs=3
  To Workspace9 : ToWorkspace  VariableName=ess_current  SampleTime=-1
  Voc-I*R : Fcn  Expr=u[2]-u[1]*u[3]
  ess max voltage*#batts : Constant  Value=ess_max_volts*ess_module_num
  iabs min=(Voc-Vmax)/R : Fcn  Expr=(u(1)-u(2))/u(3)
  limit current based on  max voltage during charge : Switch  Threshold=eps  SaturateOnIntegerOverflow=on  InputSameDT=on
  min charge current not exceeded : RelationalOperator  Operator=>  InputSameDT=on
  I_ : Outport  InitialOutput=0
  V_ : Outport  Port=2  InitialOutput=0
  tag scope: ess_maxV_limited=global
  wires:
  Logical Operator1/1 -> [ess_maxV_limited]
  ess max voltage*#batts/1 -> Mux5/2
  Mux5/1 -> iabs min=(Voc-Vmax)/R/1
  Mux4/1 -> Ibty=(Voc-(Voc^2-4RPbty)^.5)        ----------------------------- (2*R)/1
  Voc-I*R/1 -> V_/1
  Mux3/1 -> Voc-I*R/1
  min charge current not exceeded/1 -> Logical Operator1/1, limit current based on  max voltage during charge/2
  limit current based on  max voltage during charge/1 -> Mux3/1, To Workspace9/1, I_/1
  iabs min=(Voc-Vmax)/R/1 -> limit current based on  max voltage during charge/3, min charge current not exceeded/2
  Ibty=(Voc-(Voc^2-4RPbty)^.5)        ----------------------------- (2*R)/1 -> limit current based on  max voltage during charge/1, min charge current not exceeded/1
  Rint/1 -> Mux5/3, Mux3/3, Mux4/3
  Voc/1 -> Mux5/1, Mux3/2, Mux4/2
  limited output power (W)/1 -> Mux4/1

== system lib_energy_storage/Ess Choices/energy storage <ess>/documentation9 ==

== system lib_energy_storage/Ess Choices/energy storage <ess>/ess tmp ==
  Qess_gen : Inport
  Enable : EnablePort  StatesWhenEnabling=reset
  #of mods : Gain  Gain=ess_module_num  SaturateOnIntegerOverflow=on  OutDataTypeStr=Inherit: Same as input  ParamDataTypeStr=Inherit: Same as input
  1/#of mods : Gain  Gain=1/ess_module_num  SaturateOnIntegerOverflow=on  OutDataTypeStr=Inherit: Same as input  ParamDataTypeStr=Inherit: Same as input
  1/mcp : Gain  Gain=1/(ess_module_mass*ess_mod_cp)  SaturateOnIntegerOverflow=on  OutDataTypeStr=Inherit: Same as input  ParamDataTypeStr=Inherit: Same as input
  Block NOTES : Subsystem
      mask Display: disp('Block\nNOTES')
  Memory : Memory  X0=cyc_mph(1,2)*.447
  Memory1 : Memory  X0=cyc_mph(1,2)*.447
  Mux20 : Mux  Inputs=3
  Qc : Sum  SaturateOnIntegerOverflow=on  InputSameDT=on  OutDataTypeStr=Inherit: Same as first input
  Qess_case : Fcn  Expr=(u(2) - u(1))/u(3)
  Saturation3 : Saturate  UpperLimit=1  LowerLimit=0
  Tair,ave : Subsystem  TreatAsAtomicUnit=on
  Tess2 : Integrator  InitialCondition=ess_mod_init_tmp
  thermostat : Fcn  Expr=u(1) - ess_set_tmp
  Tess : Outport  InitialOutput=0
  Tair : Outport  Port=2
  Qair : Outport  Port=3  OutputWhenDisabled=reset  InitialOutput=0
  wires:
  Tair,ave/2(Th Res) -> Mux20/3
  Mux20/1 -> Qess_case/1
  #of mods/1 -> Qair/1
  Memory/1 -> Tair,ave/1(Qess_case), Tair,ave/2(Qess_case1)
  Memory1/1 -> Tair,ave/Enable
  Saturation3/1 -> Memory1/1
  thermostat/1 -> Saturation3/1
  1/#of mods/1 -> Qc/2
  Qess_gen/1 -> 1/#of mods/1
  Tess2/1 -> thermostat/1, Mux20/1, Tess/1
  1/mcp/1 -> Tess2/1
  Qess_case/1 -> #of mods/1, Memory/1, Qc/1
  Qc/1 -> 1/mcp/1
  Tair,ave/3(Tair) -> Tair/1
  Tair,ave/1(Tair_ave) -> Mux20/2

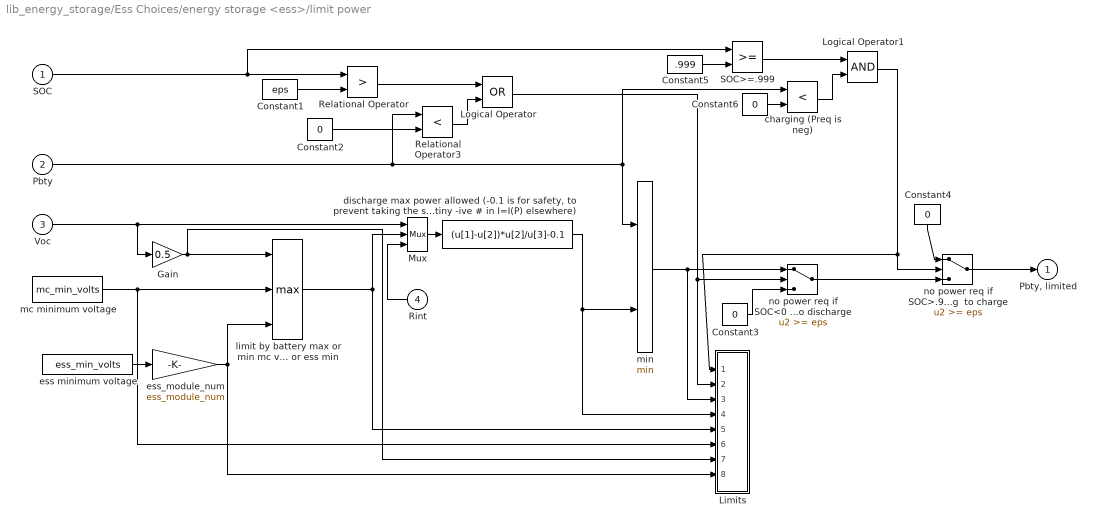
== system lib_energy_storage/Ess Choices/energy storage <ess>/limit power ==
  SOC : Inport
  Pbty : Inport  Port=2
  Voc : Inport  Port=3
  Rint : Inport  Port=4
  Constant1 : Constant  Value=eps
  Constant{2..4,6} (4 alike) : Constant  Value=0
  Constant5 : Constant  Value=.999
  Gain : Gain  Gain=0.5  SaturateOnIntegerOverflow=on  OutDataTypeStr=Inherit: Same as input  ParamDataTypeStr=Inherit: Same as input
  Limits : Subsystem
  Logical Operator : Logic  Operator=OR
  Logical Operator1 : Logic
  Mux : Mux  Inputs=3
  Relational Operator : RelationalOperator  Operator=>  InputSameDT=on
  Relational Operator3 : RelationalOperator  Operator=<  InputSameDT=on
  SOC>=.999 : RelationalOperator  InputSameDT=on
  charging (Preq is neg) : RelationalOperator  Operator=<  InputSameDT=on
  "discharge max power allowed (-0.1 is for safety, to prevent taking the square of a tiny -ive # in I=I(P) elsewhere)" : Fcn  Expr=(u[1]-u[2])*u[2]/u[3]-0.1
  ess minimum voltage : Constant  Value=ess_min_volts
  ess_module_num : Gain  Gain=ess_module_num  SaturateOnIntegerOverflow=on  OutDataTypeStr=Inherit: Same as input  ParamDataTypeStr=Inherit: Same as input
  limit by battery max or min mc voltage or ess min : MinMax  Function=max  Inputs=3  SaturateOnIntegerOverflow=on  InputSameDT=on
  mc minimum voltage : Constant  Value=mc_min_volts
  min : MinMax  Inputs=2  SaturateOnIntegerOverflow=on  InputSameDT=on
  no power req if SOC<0 and trying  to discharge : Switch  Threshold=eps  SaturateOnIntegerOverflow=on  InputSameDT=on
  no power req if SOC>.999 and trying  to charge : Switch  Threshold=eps  SaturateOnIntegerOverflow=on  InputSameDT=on
  "Pbty, limited" : Outport  InitialOutput=0
  wires:
  Logical Operator1/1 -> Limits/1(SOC  high limited), no power req if SOC>.999 and trying  to charge/2
  no power req if SOC>.999 and trying  to charge/1 -> "Pbty, limited"/1
  no power req if SOC<0 and trying  to discharge/1 -> no power req if SOC>.999 and trying  to charge/3
  Constant4/1 -> no power req if SOC>.999 and trying  to charge/1
  Constant5/1 -> SOC>=.999/2
  charging (Preq is neg)/1 -> Logical Operator1/2
  Constant6/1 -> charging (Preq is neg)/2
  SOC>=.999/1 -> Logical Operator1/1
  SOC/1 -> SOC>=.999/1, Relational Operator/1
  ess_module_num/1 -> Limits/8(V ess_min_volts), limit by battery max or min mc voltage or ess min/3
  ess minimum voltage/1 -> ess_module_num/1
  Gain/1 -> Limits/7(V battery (.5Voc)), limit by battery max or min mc voltage or ess min/1
  Rint/1 -> Mux/3
  mc minimum voltage/1 -> Limits/6(V mc_min_volts), limit by battery max or min mc voltage or ess min/2
  "discharge max power allowed (-0.1 is for safety, to prevent taking the square of a tiny -ive # in I=I(P) elsewhere)"/1 -> min/2, Limits/4(power bat limited)
  limit by battery max or min mc voltage or ess min/1 -> Limits/5(V used), Mux/2
  Mux/1 -> "discharge max power allowed (-0.1 is for safety, to prevent taking the square of a tiny -ive # in I=I(P) elsewhere)"/1
  min/1 -> Limits/3(power req), no power req if SOC<0 and trying  to discharge/1
  Voc/1 -> Gain/1, Mux/1
  Logical Operator/1 -> Limits/2(not SOC  low limited), no power req if SOC<0 and trying  to discharge/2
  Constant3/1 -> no power req if SOC<0 and trying  to discharge/3
  Relational Operator3/1 -> Logical Operator/2
  Constant2/1 -> Relational Operator3/2
  Pbty/1 -> charging (Preq is neg)/1, min/1, Relational Operator3/1
  Relational Operator/1 -> Logical Operator/1
  Constant1/1 -> Relational Operator/2
